simulink model "Simulink_Cont_Sys_Q4"  (R2022b)
settings: Solver=VariableStepAuto  StartTime=0.0  StopTime=25  RelTol=1e-3
libraries: cstblocks x2
settings Model: Creator=user  LastModifiedBy=user

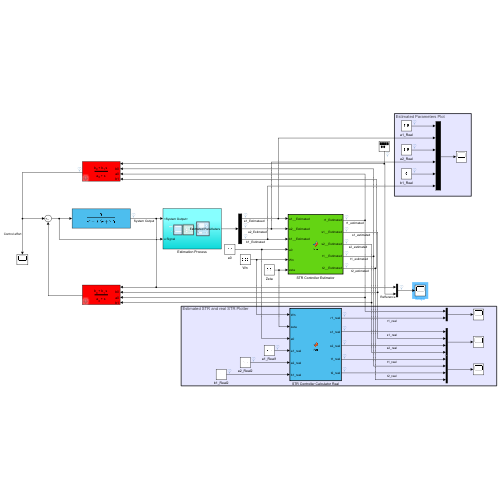
[thumbnail: Simulink's stored preview of the top-level diagram]
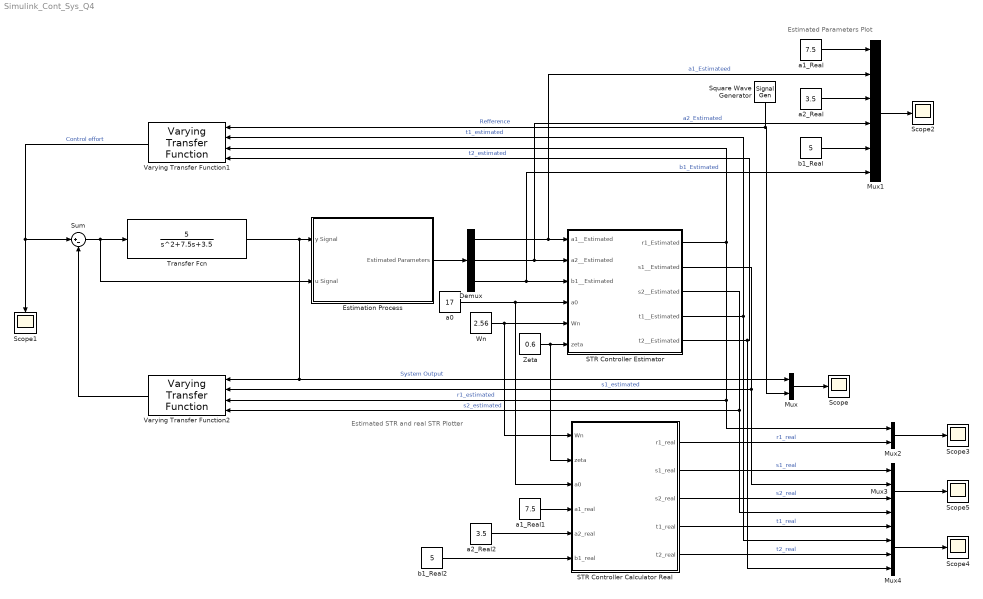
== system Simulink_Cont_Sys_Q4 ==
  note: Estimated STR and real STR Plotter
  note: Estimated Parameters Plot
  Demux : Demux  Outputs=3
  Estimation Process : Subsystem
  Mux : Mux  Inputs=2
  Mux1 : Mux  Inputs=6
  Mux2 : Mux  Inputs=2
  Mux3 : Mux
  Mux4 : Mux
  STR Controller Calculator Real : MATLAB Function  TreatAsAtomicUnit=on
  STR Controller Estimator : MATLAB Function  TreatAsAtomicUnit=on
  Scope{,1..5} (6 alike) : Scope
  Square Wave Generator : SignalGenerator  WaveForm=square  Frequency=0.08
  Sum : Sum  Inputs=|+-
  Transfer Fcn : TransferFcn  Numerator=[5]  Denominator=[1 7.5 3.5]
  Varying Transfer Function1 : cstblocks/Linear Parameter Varying/Varying Transfer Function  N=1
  Varying Transfer Function2 : cstblocks/Linear Parameter Varying/Varying Transfer Function  N=1
  Wn : Constant  Value=2.56
  Zeta : Constant  Value=0.6
  a0 : Constant  Value=17
  a1_Real : Constant  Value=7.5
  a1_Real1 : Constant  Value=7.5
  a2_Real : Constant  Value=3.5
  a2_Real2 : Constant  Value=3.5
  b1_Real : Constant  Value=5
  b1_Real2 : Constant  Value=5
  wires:
  Transfer Fcn/1 -> Varying Transfer Function2/1, Mux/1, Estimation Process/1(" y Signal")  "System Output"
  Square Wave Generator/1 -> Mux/2, Varying Transfer Function1/1  "Refference"
  Varying Transfer Function1/1 -> Sum/1, Scope1/1  "Control effort"
  Sum/1 -> Estimation Process/2(u Signal), Transfer Fcn/1
  Estimation Process/1(Estimated Parameters) -> Demux/1
  Demux/1 -> Mux1/2, STR Controller Estimator/1(a1__Estimated)  "a1_Estimateed"
  Demux/2 -> STR Controller Estimator/2(a2__Estimated), Mux1/4  "a2_Estimated"
  Demux/3 -> STR Controller Estimator/3(b1__Estimated), Mux1/6  "b1_Estimated"
  a0/1 -> STR Controller Calculator Real/3(a0), STR Controller Estimator/4(a0)
  STR Controller Estimator/1(r1_Estimated) -> Mux2/1, Varying Transfer Function2/3, Varying Transfer Function1/3  "r1_estimated"
  STR Controller Estimator/2(s1__Estimated) -> Mux3/2, Varying Transfer Function2/2  "s1_estimated"
  STR Controller Estimator/3(s2__Estimated) -> Varying Transfer Function2/4, Mux3/4  "s2_estimated"
  STR Controller Estimator/4(t1__Estimated) -> Varying Transfer Function1/2, Mux4/2  "t1_estimated"
  STR Controller Estimator/5(t2__Estimated) -> Mux4/4, Varying Transfer Function1/4  "t2_estimated"
  Varying Transfer Function2/1 -> Sum/2
  Mux/1 -> Scope/1
  Wn/1 -> STR Controller Calculator Real/1(Wn), STR Controller Estimator/5(Wn)
  Zeta/1 -> STR Controller Calculator Real/2(zeta), STR Controller Estimator/6(zeta)
  a1_Real/1 -> Mux1/1
  a2_Real/1 -> Mux1/3
  b1_Real/1 -> Mux1/5
  Mux1/1 -> Scope2/1
  a1_Real1/1 -> STR Controller Calculator Real/4(a1_real)
  a2_Real2/1 -> STR Controller Calculator Real/5(a2_real)
  b1_Real2/1 -> STR Controller Calculator Real/6(b1_real)
  STR Controller Calculator Real/1(r1_real) -> Mux2/2  "r1_real"
  STR Controller Calculator Real/2(s1_real) -> Mux3/1  "s1_real"
  STR Controller Calculator Real/3(s2_real) -> Mux3/3  "s2_real"
  STR Controller Calculator Real/4(t1_real) -> Mux4/1  "t1_real"
  STR Controller Calculator Real/5(t2_real) -> Mux4/3  "t2_real"
  Mux2/1 -> Scope3/1
  Mux3/1 -> Scope5/1
  Mux4/1 -> Scope4/1

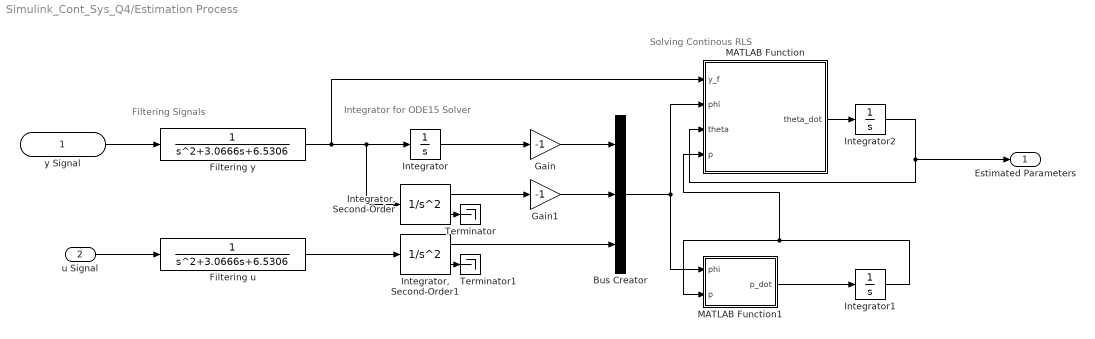
== system Simulink_Cont_Sys_Q4/Estimation Process ==
  note: Solving Continous RLS
  note: Integrator for ODE15 Solver
  note: Filtering Signals
  " y Signal" : Inport
  u Signal : Inport  Port=2
  Bus Creator : BusCreator  Inputs=3
  Filtering u : TransferFcn  Denominator=[1 3.0666 6.5306]
  Filtering y : TransferFcn  Denominator=[1 3.0666 6.5306]
  Gain : Gain  Gain=-1
  Gain1 : Gain  Gain=-1
  Integrator : Integrator
  "Integrator, Second-Order" : SecondOrderIntegrator
  "Integrator, Second-Order1" : SecondOrderIntegrator
  Integrator1 : Integrator  InitialCondition=100000*eye(3)
  Integrator2 : Integrator  InitialCondition=[2 2 2]
  MATLAB Function : MATLAB Function  TreatAsAtomicUnit=on
  MATLAB Function1 : MATLAB Function  TreatAsAtomicUnit=on
  Terminator : Terminator
  Terminator1 : Terminator
  Estimated Parameters : Outport
  wires:
  Gain1/1 -> Bus Creator/2
  Bus Creator/1 -> MATLAB Function1/1(phi), MATLAB Function/2(phi)
  Filtering y/1 -> MATLAB Function/1(y_f), "Integrator, Second-Order"/1, Integrator/1
  Integrator/1 -> Gain/1
  "Integrator, Second-Order1"/2 -> Terminator1/1
  "Integrator, Second-Order1"/1 -> Bus Creator/3
  Integrator1/1 -> MATLAB Function/4(p), MATLAB Function1/2(p)
  Filtering u/1 -> "Integrator, Second-Order1"/1
  "Integrator, Second-Order"/2 -> Terminator/1
  MATLAB Function/1(theta_dot) -> Integrator2/1
  "Integrator, Second-Order"/1 -> Gain1/1
  Gain/1 -> Bus Creator/1
  " y Signal"/1 -> Filtering y/1
  Integrator2/1 -> Estimated Parameters/1, MATLAB Function/3(theta)
  u Signal/1 -> Filtering u/1
  MATLAB Function1/1(p_dot) -> Integrator1/1

== matlab function Simulink_Cont_Sys_Q4/Estimation Process/MATLAB Function1 ==
  data: phi input; p_dot output; p input
function p_dot = fcn(phi,p)
alpha = 1.0 ;
p_dot = alpha*p - p*(phi)*(phi)'*p ;

== matlab function Simulink_Cont_Sys_Q4/Estimation Process/MATLAB Function ==
  data: y_f input; theta_dot output; phi input; theta input; p input
function theta_dot = fcn(y_f,phi,theta,p)
theta_dot = (p)*(phi)*(y_f-(phi')*theta);

== matlab function Simulink_Cont_Sys_Q4/STR Controller Estimator ==
  data: a1__Estimated input; a2__Estimated input; b1__Estimated input; a0 input; Wn input; r1_Estimated output; zeta input; s1__Estimated output; s2__Estimated output; t1__Estimated output; t2__Estimated output
function [r1_Estimated,s1__Estimated,s2__Estimated,t1__Estimated,t2__Estimated] = fcn(a1__Estimated,a2__Estimated,b1__Estimated,a0,Wn,zeta)
r1_Estimated = 2*zeta*Wn+a0-a1__Estimated ;
s1__Estimated = (Wn^2+2*a0*zeta*Wn-a1__Estimated*r1_Estimated-a2__Estimated)/b1__Estimated ;
s2__Estimated = (Wn^2*a0-a2__Estimated*r1_Estimated)/(b1__Estimated) ;
t1__Estimated = Wn^2/b1__Estimated ;
t2__Estimated = Wn^2*a0/b1__Estimated ;

== matlab function Simulink_Cont_Sys_Q4/STR Controller Calculator Real ==
  data: Wn input; r1_real output; zeta input; a0 input; a1_real input; a2_real input; b1_real input; s1_real output; s2_real output; t1_real output; t2_real output
function [r1_real,s1_real,s2_real,t1_real,t2_real] = fcn(Wn,zeta,a0,a1_real,a2_real,b1_real)

r1_real = 2*zeta*Wn+a0-a1_real ;
s1_real = (Wn^2+2*a0*zeta*Wn-a1_real*r1_real-a2_real)/b1_real ;
s2_real = (Wn^2*a0-a2_real*r1_real)/(b1_real) ;
t1_real = Wn^2/b1_real ;
t2_real = Wn^2*a0/b1_real ;
